simulink model "linear_speed_control_R2015a"  (R2015b)
settings: Solver=ode45  StartTime=0.0  StopTime=10.0  RelTol=1e-3
values from neighbouring files (symbols this model uses):
  gamma_com = 1*pi/180    (= 0.0174532925199)    [RunSimLab7.m]    (also in RunSimLab7[Conflict].m = 0.0349065850399)
  kdg = 1    [RunSimLab7.m]    (also in RunSimLab7[Conflict].m = [.4])
  kdu = [0]    [RunSimLab7.m]    (also in RunSimLab7[Conflict].m)
  kig = 1    [RunSimLab7.m]    (also in RunSimLab7[Conflict].m = [.2])
  kiu = [0]    [RunSimLab7.m]    (also in RunSimLab7[Conflict].m = [.5])
  kpg = 1    [RunSimLab7.m]    (also in RunSimLab7[Conflict].m = [1])
  kpu = [0]    [RunSimLab7.m]    (also in RunSimLab7[Conflict].m = [.3])
  numP_gamma_from_de = numPde(4,:)-numPde(2,:)/V_trim    [RunSimLab7[Conflict].m]
  numP_gamma_from_dt = numPdt(4,:)-numPdt(2,:)/V_trim    [RunSimLab7[Conflict].m]
  numP_u_from_de = numPde(1,:)    [RunSimLab7[Conflict].m]
  numP_u_from_dt = numPdt(1,:)    [RunSimLab7[Conflict].m]
  u_com = 1    [RunSimLab7.m]    (also in RunSimLab7[Conflict].m)
undefined symbols (not defined in the file or in its folder): denPde, denPdt
settings Model: Creator=Eric  LastModifiedBy=Jeremy
settings DataIOCC: SaveFormat=Array  SaveState=on
settings OptimizationCC: ExpressionDepthLimit=2147483647
settings DebuggingCC: UnderspecifiedInitializationDetection=Classic  MergeDetectMultiDrivingBlocksExec=none  SolverPrmCheckMsg=warning  StateNameClashWarn=warning
settings HardwareCC: ProdBitPerPointer=32  ProdLargestAtomicFloat=None  ProdIntDivRoundTo=Undefined  ProdEndianess=Unspecified  ProdWordSize=32  ProdHWDeviceType=32-bit Generic
settings GRTTargetCC: GeneratePreprocessorConditionals=Disable all
settings ConfigComp: CovModelRefEnable=Off  CovSFcnEnable=off

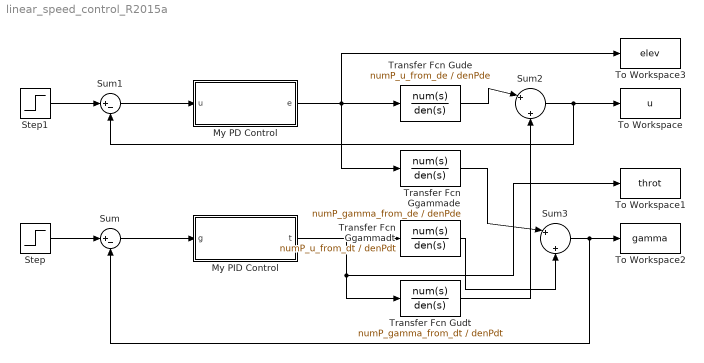
== system linear_speed_control_R2015a ==
  My PD Control : Subsystem  TreatAsAtomicUnit=on
  My PID Control : Subsystem  TreatAsAtomicUnit=on
  Step : Step  Time=0  After=u_com  SampleTime=0
  Step1 : Step  Time=0  After=gamma_com  SampleTime=0
  Sum : Sum  Inputs=|+-
  Sum1 : Sum  Inputs=|+-
  Sum2 : Sum  Inputs=|+|+
  Sum3 : Sum  Inputs=|+|+
  To Workspace : ToWorkspace  VariableName=u  SaveFormat=Timeseries  SampleTime=-1
  To Workspace1 : ToWorkspace  VariableName=throt  SaveFormat=Timeseries  SampleTime=-1
  To Workspace2 : ToWorkspace  VariableName=gamma  SaveFormat=Timeseries  SampleTime=-1
  To Workspace3 : ToWorkspace  VariableName=elev  SaveFormat=Timeseries  SampleTime=-1
  Transfer Fcn Ggammade : TransferFcn  Numerator=numP_gamma_from_de  Denominator=denPde
  Transfer Fcn Ggammadt : TransferFcn  Numerator=numP_u_from_dt  Denominator=denPdt
  Transfer Fcn Gude : TransferFcn  Numerator=numP_u_from_de  Denominator=denPde
  Transfer Fcn Gudt : TransferFcn  Numerator=numP_gamma_from_dt  Denominator=denPdt
  wires:
  Step/1 -> Sum/1
  Sum/1 -> My PID Control/1(g)
  My PID Control/1(t) -> Transfer Fcn Gudt/1, To Workspace1/1, Transfer Fcn Ggammadt/1
  Sum1/1 -> My PD Control/1(u)
  My PD Control/1(e) -> To Workspace3/1, Transfer Fcn Ggammade/1, Transfer Fcn Gude/1
  Step1/1 -> Sum1/1
  Transfer Fcn Ggammade/1 -> Sum3/1
  Transfer Fcn Ggammadt/1 -> Sum3/2
  Sum3/1 -> Sum/2, To Workspace2/1
  Transfer Fcn Gudt/1 -> Sum2/2
  Transfer Fcn Gude/1 -> Sum2/1
  Sum2/1 -> Sum1/2, To Workspace/1

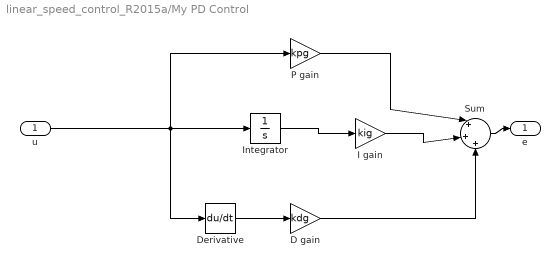
== system linear_speed_control_R2015a/My PD Control ==
  u : Inport
  D gain : Gain  Gain=kdg
  Derivative : Derivative
  I gain : Gain  Gain=kig
  Integrator : Integrator
  P gain : Gain  Gain=kpg
  Sum : Sum  Inputs=|+|+|+
  e : Outport
  wires:
  u/1 -> Derivative/1, Integrator/1, P gain/1
  P gain/1 -> Sum/1
  Sum/1 -> e/1
  Derivative/1 -> D gain/1
  Integrator/1 -> I gain/1
  D gain/1 -> Sum/3
  I gain/1 -> Sum/2

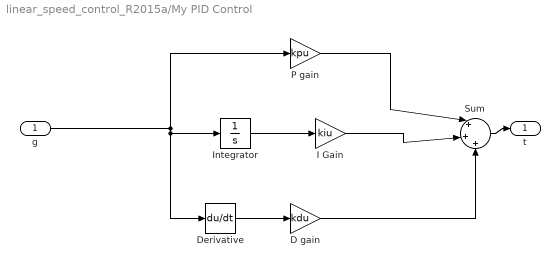
== system linear_speed_control_R2015a/My PID Control ==
  g : Inport
  D gain : Gain  Gain=kdu
  Derivative : Derivative
  I Gain : Gain  Gain=kiu
  Integrator : Integrator
  P gain : Gain  Gain=kpu
  Sum : Sum  Inputs=|+|+|+
  t : Outport
  wires:
  g/1 -> Integrator/1, Derivative/1, P gain/1
  P gain/1 -> Sum/1
  Sum/1 -> t/1
  Derivative/1 -> D gain/1
  Integrator/1 -> I Gain/1
  D gain/1 -> Sum/3
  I Gain/1 -> Sum/2
